simulink library "WBToolboxLibrary"  (R2014b)
settings: Solver=ode45  StartTime=0.0  StopTime=10.0  RelTol=1e-3
undefined symbols (not defined in the file): WBT_modelName, WBT_robotName, WBT_wbiFilename, WBT_wbiList
libraries: simulink x1
(part 2 of 2)

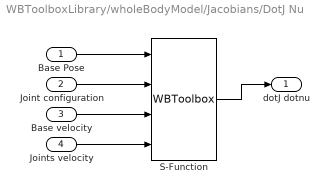
== system WBToolboxLibrary/wholeBodyModel/Jacobians/DotJ Nu ==
  Base Pose : Inport
  Joint configuration : Inport  Port=2
  Base velocity : Inport  Port=3
  Joints velocity : Inport  Port=4
  S-Function : S-Function  FunctionName=WBToolbox  Parameters='DotJNu',robotName,localName,wbiFile,wbiList,frameName  SFunctionDeploymentMode=off  EnableBusSupport=off
  dotJ dotnu : Outport
  wires:
  Joint configuration/1 -> S-Function/2
  Base Pose/1 -> S-Function/1
  S-Function/1 -> dotJ dotnu/1
  Base velocity/1 -> S-Function/3
  Joints velocity/1 -> S-Function/4

== system WBToolboxLibrary/wholeBodyModel/Jacobians/Jacobian ==
  Base Pose : Inport
  Joint configuration : Inport  Port=2
  S-Function : S-Function  FunctionName=WBToolbox  Parameters='Jacobian',robotName,localName,wbiFile,wbiList,frameName  SFunctionDeploymentMode=off  EnableBusSupport=off
  Forward Kinematics : Outport
  wires:
  S-Function/1 -> Forward Kinematics/1
  Base Pose/1 -> S-Function/1
  Joint configuration/1 -> S-Function/2

== system WBToolboxLibrary/wholeBodyModel/Kinematics/Forward Kinematics ==
  Base Pose : Inport
  Joint configuration : Inport  Port=2
  S-Function : S-Function  FunctionName=WBToolbox  Parameters='ForwardKinematics',robotName,localName,wbiFile,wbiList,frameName  SFunctionDeploymentMode=off  EnableBusSupport=off
  Forward Kinematics : Outport
  wires:
  S-Function/1 -> Forward Kinematics/1
  Base Pose/1 -> S-Function/1
  Joint configuration/1 -> S-Function/2

== system WBToolboxLibrary/wholeBodyModel/Kinematics/Inverse Kinematics ==
  Desired frame pose : Inport
  Current Base Pose : Inport  Port=2
  Current Joint configuration : Inport  Port=3
  S-Function : S-Function  FunctionName=WBToolbox  Parameters='InverseKinematics',robotName,localName,wbiFile,wbiList,robotPart,optOption  SFunctionDeploymentMode=off  EnableBusSupport=off
  Desired Base Pose : Outport
  Desired Joint Configuration : Outport  Port=2
  wires:
  S-Function/1 -> Desired Base Pose/1
  Current Base Pose/1 -> S-Function/2
  Current Joint configuration/1 -> S-Function/3
  Desired frame pose/1 -> S-Function/1
  S-Function/2 -> Desired Joint Configuration/1

== matlab function WBToolboxLibrary/Utilities/holder /MATLAB Function ==
  data: s input; s0 output; unused input
function s0 = fcn(s, ~)
persistent state
%#codegen

if isempty(state)
    state = s;
end

s0 = state;

== matlab function WBToolboxLibrary/Utilities/DampPinv/Damped Pseudo Inverse ==
  data: mat input; DPinv output; sigma input
function DPinv  = fcn(mat,sigma)
% Economody size svd of mat
[U,S,V] = svd(mat,'econ');
% Damped version of S with sigma
S(S>sigma)=S(S>sigma)./((S(S>sigma)).^2+sigma^2);
% Damped pseudoinverse
DPinv = V*pinv(S)*U';

== matlab function WBToolboxLibrary/Utilities/TruncPinv/Truncated PseudoInverse ==
  data: mat input; TPinv output; tol input
function TPinv  = fcn(mat,tol)
%#codegen
[U,S,V] = svd(mat,'econ');
% Setting to zero value
% Setting to 1/S(i,i) singular values greater than tol
 S(S>tol)=1./S(S>tol);
 TPinv = V*pinv(S)*U';
